simulink model "SWC_FDC_type"  (R2021b)
settings: Solver=FixedStepDiscrete  StartTime=0.0  StopTime=10.0  FixedStep=0.001  RelTol=1e-3
values from neighbouring files (symbols this model uses):
  C_TASK_5MS_S = (	C_TICK_TIME_S      	)    [vcu_local_hdr.m]
  DID_VCUKey = uint16(0x0202)    [vcu_local_hdr.m]
  DID_XWD = uint16(513)    [vcu_local_hdr.m]
  DIDLen_APPPedalZP = uint16(3)    [vcu_local_hdr.m]
  DIDLen_APSFunConfig = uint16(16)    [vcu_local_hdr.m]
  DIDLen_AutoLock = uint16(1)    [vcu_local_hdr.m]
  DIDLen_AutoWipHSpdEN = uint16(1)    [vcu_local_hdr.m]
  DIDLen_DKCKey = uint16(8)    [vcu_local_hdr.m]
  DIDLen_DRLDis = uint16(1)    [vcu_local_hdr.m]
  DIDLen_DynoMode = uint16(1)    [vcu_local_hdr.m]
  DIDLen_FMHTimer = uint16(1)    [vcu_local_hdr.m]
  DIDLen_LFLowPresThre = uint16(1)    [vcu_local_hdr.m]
  DIDLen_LFSensorID = uint16(4)    [vcu_local_hdr.m]
  DIDLen_LRLowPresThre = uint16(1)    [vcu_local_hdr.m]
  DIDLen_LRSensorID = uint16(4)    [vcu_local_hdr.m]
  DIDLen_NVMPedalZP = uint16(3)    [vcu_local_hdr.m]
  DIDLen_RFLowPresThre = uint16(1)    [vcu_local_hdr.m]
  DIDLen_RFSensorID = uint16(4)    [vcu_local_hdr.m]
  DIDLen_RRLowPresThre = uint16(1)    [vcu_local_hdr.m]
  DIDLen_RRSensorID = uint16(4)    [vcu_local_hdr.m]
  DIDLen_SensorMode = uint16(1)    [vcu_local_hdr.m]
  DIDLen_TireSize = uint16(16)    [vcu_local_hdr.m]
  DIDLen_TPMSLearnSta = uint16(1)    [vcu_local_hdr.m]
  DIDLen_TurnLampFLThreCurr = uint16(1)    [vcu_local_hdr.m]
  DIDLen_TurnLampFRThreCurr = uint16(1)    [vcu_local_hdr.m]
  DIDLen_TurnLampRLThreCurr = uint16(1)    [vcu_local_hdr.m]
  DIDLen_TurnLampRRThreCurr = uint16(1)    [vcu_local_hdr.m]
  DIDLen_USSConfig = uint16(16)    [vcu_local_hdr.m]
  DIDLen_WhlPres = uint16(4)    [vcu_local_hdr.m]
  DIDLen_WhlSensorBattSta = uint16(1)    [vcu_local_hdr.m]
  DIDLen_WhlTmp = uint16(4)    [vcu_local_hdr.m]
  DIDLen_WipRLSCmdCutFilter = uint16(1)    [vcu_local_hdr.m]
  DIDLen_WipRLSCmdHoldFilter = uint16(1)    [vcu_local_hdr.m]
  DIDLen_XWDMode = uint16(1)    [vcu_local_hdr.m]
  DIDNum_APPPedalZP = uint16(0x0206)    [vcu_local_hdr.m]
  DIDNum_APSFunConfig = uint16(0x0903)    [vcu_local_hdr.m]
  DIDNum_AutoLock = uint16(0x0306)    [vcu_local_hdr.m]
  DIDNum_AutoWipHSpdEN = uint16(0x0308)    [vcu_local_hdr.m]
  DIDNum_DKCKey = uint16(0x0202)    [vcu_local_hdr.m]
  DIDNum_DRLDis = uint16(0x0307)    [vcu_local_hdr.m]
  DIDNum_DynoMode = uint16(0x0203)    [vcu_local_hdr.m]
  DIDNum_FMHTimer = uint16(0x0305)    [vcu_local_hdr.m]
  DIDNum_LFLowPresThre = uint16(0x0B08)    [vcu_local_hdr.m]
  DIDNum_LFSensorID = uint16(0x0B01)    [vcu_local_hdr.m]
  DIDNum_LRLowPresThre = uint16(0x0B0A)    [vcu_local_hdr.m]
  DIDNum_LRSensorID = uint16(0x0B03)    [vcu_local_hdr.m]
  DIDNum_NVMPedalZP = uint16(0x0207)    [vcu_local_hdr.m]
  DIDNum_RFLowPresThre = uint16(0x0B09)    [vcu_local_hdr.m]
  DIDNum_RFSensorID = uint16(0x0B02)    [vcu_local_hdr.m]
  DIDNum_RRLowPresThre = uint16(0x0B0B)    [vcu_local_hdr.m]
  DIDNum_RRSensorID = uint16(0x0B04)    [vcu_local_hdr.m]
  DIDNum_SensorMode = uint16(0x0B0C)    [vcu_local_hdr.m]
  DIDNum_TireSize = uint16(0x0902)    [vcu_local_hdr.m]
  DIDNum_TPMSLearnSta = uint16(0x0B0D)    [vcu_local_hdr.m]
  DIDNum_TurnLampFLThreCurr = uint16(0x0303)    [vcu_local_hdr.m]
  DIDNum_TurnLampFRThreCurr = uint16(0x0301)    [vcu_local_hdr.m]
  DIDNum_TurnLampRLThreCurr = uint16(0x0304)    [vcu_local_hdr.m]
  DIDNum_TurnLampRRThreCurr = uint16(0x0302)    [vcu_local_hdr.m]
  DIDNum_USSConfig = uint16(0x0901)    [vcu_local_hdr.m]
  DIDNum_WhlPres = uint16(0x0B05)    [vcu_local_hdr.m]
  DIDNum_WhlSensorBattSta = uint16(0x0B07)    [vcu_local_hdr.m]
  DIDNum_WhlTmp = uint16(0x0B06)    [vcu_local_hdr.m]
  DIDNum_WipRLSCmdCutFilter = uint16(0x030A)    [vcu_local_hdr.m]
  DIDNum_WipRLSCmdHoldFilter = uint16(0x0309)    [vcu_local_hdr.m]
  DIDNum_XWDMode = uint16(0x0201)    [vcu_local_hdr.m]
  DIDVCUKeyLength = uint16(8)    [vcu_local_hdr.m]
  DTC_10020B = Simulink.Parameter    [DTC_Constant_Definition.m]
  DTC_10020C = Simulink.Parameter    [DTC_Constant_Definition.m]
  DTC_10020D = Simulink.Parameter    [DTC_Constant_Definition.m]
  DTC_10020E = Simulink.Parameter    [DTC_Constant_Definition.m]
  DTC_100210 = Simulink.Parameter    [DTC_Constant_Definition.m]
  DTC_100211 = Simulink.Parameter    [DTC_Constant_Definition.m]
  DTC_100212 = Simulink.Parameter    [DTC_Constant_Definition.m]
  DTC_100213 = Simulink.Parameter    [DTC_Constant_Definition.m]
  DTC_100214 = Simulink.Parameter    [DTC_Constant_Definition.m]
  DTC_100215 = Simulink.Parameter    [DTC_Constant_Definition.m]
  DTC_100216 = Simulink.Parameter    [DTC_Constant_Definition.m]
  DTC_100217 = Simulink.Parameter    [DTC_Constant_Definition.m]
  DTC_100218 = Simulink.Parameter    [DTC_Constant_Definition.m]
  DTC_100219 = Simulink.Parameter    [DTC_Constant_Definition.m]
  DTC_10021A = Simulink.Parameter    [DTC_Constant_Definition.m]
  DTC_10021B = Simulink.Parameter    [DTC_Constant_Definition.m]
  DTC_10021C = Simulink.Parameter    [DTC_Constant_Definition.m]
  DTC_10021D = Simulink.Parameter    [DTC_Constant_Definition.m]
  DTC_10021E = Simulink.Parameter    [DTC_Constant_Definition.m]
  DTC_100220 = Simulink.Parameter    [DTC_Constant_Definition.m]
  DTC_100221 = Simulink.Parameter    [DTC_Constant_Definition.m]
  DTC_100223 = Simulink.Parameter    [DTC_Constant_Definition.m]
  DTC_100224 = Simulink.Parameter    [DTC_Constant_Definition.m]
  DTC_100225 = Simulink.Parameter    [DTC_Constant_Definition.m]
  DTC_100226 = Simulink.Parameter    [DTC_Constant_Definition.m]
  DTC_100227 = Simulink.Parameter    [DTC_Constant_Definition.m]
  DTC_100242 = Simulink.Parameter    [DTC_Constant_Definition.m]
  DTC_100243 = Simulink.Parameter    [DTC_Constant_Definition.m]
  DTC_100244 = Simulink.Parameter    [DTC_Constant_Definition.m]
  DTC_100247 = Simulink.Parameter    [DTC_Constant_Definition.m]
  DTC_100248 = Simulink.Parameter    [DTC_Constant_Definition.m]
  DTC_100249 = Simulink.Parameter    [DTC_Constant_Definition.m]
  DTC_100250 = Simulink.Parameter    [DTC_Constant_Definition.m]
  DTC_100251 = Simulink.Parameter    [DTC_Constant_Definition.m]
  DTC_100252 = Simulink.Parameter    [DTC_Constant_Definition.m]
  DTC_100A10 = Simulink.Parameter    [DTC_Constant_Definition.m]
  DTC_100A12 = Simulink.Parameter    [DTC_Constant_Definition.m]
  DTC_100A16 = Simulink.Parameter    [DTC_Constant_Definition.m]
  DTC_100A17 = Simulink.Parameter    [DTC_Constant_Definition.m]
  DTC_100A18 = Simulink.Parameter    [DTC_Constant_Definition.m]
  DTC_100A19 = Simulink.Parameter    [DTC_Constant_Definition.m]
  DTC_500B01 = Simulink.Parameter    [DTC_Constant_Definition.m]
  DTC_500B02 = Simulink.Parameter    [DTC_Constant_Definition.m]
  DTC_500B03 = Simulink.Parameter    [DTC_Constant_Definition.m]
  DTC_500B04 = Simulink.Parameter    [DTC_Constant_Definition.m]
  DTC_500B05 = Simulink.Parameter    [DTC_Constant_Definition.m]
  DTC_500B06 = Simulink.Parameter    [DTC_Constant_Definition.m]
  DTC_500B07 = Simulink.Parameter    [DTC_Constant_Definition.m]
  DTC_500B08 = Simulink.Parameter    [DTC_Constant_Definition.m]
  DTC_500B09 = Simulink.Parameter    [DTC_Constant_Definition.m]
  DTC_500B0A = Simulink.Parameter    [DTC_Constant_Definition.m]
  DTC_500B0B = Simulink.Parameter    [DTC_Constant_Definition.m]
  DTC_500B0C = Simulink.Parameter    [DTC_Constant_Definition.m]
  DTC_500B0D = Simulink.Parameter    [DTC_Constant_Definition.m]
  ... (+93 more)
undefined symbols (not defined in the file or in its folder): f32_ApsOutVehSpdSig, KHAL_CANBusOffDebounce_cnt, KHAL_CANBusOffDebounce_s, KHAL_DKCDecryptEnable_flg_ovrdflg, KHAL_DKCDecryptEnable_flg_ovrdval, KHAL_RandomNumberY1_enum, KHAL_RandomNumberY2_enum, KHAL_RandomNumberY_ovrdflg, KHAL_TPMSRESBUTT_flg_ovrdflg, KHAL_TPMSRESBUTT_flg_ovrdval, KINP_ReadVinCode_flg, KTQD_DefaultRegenMode_enum, R_DIDWriteCDD_CSOP_DIDSet_APPPedalZP, R_DIDWriteCDD_CSOP_DIDSet_APSFunConfig, R_DIDWriteCDD_CSOP_DIDSet_AutoLock, R_DIDWriteCDD_CSOP_DIDSet_AutoWipHSpdEN, R_DIDWriteCDD_CSOP_DIDSet_DKCKey, R_DIDWriteCDD_CSOP_DIDSet_DRLDis, R_DIDWriteCDD_CSOP_DIDSet_DynoMode, R_DIDWriteCDD_CSOP_DIDSet_FMHTimer, R_DIDWriteCDD_CSOP_DIDSet_LFLowPresThre, R_DIDWriteCDD_CSOP_DIDSet_LFSensorID, R_DIDWriteCDD_CSOP_DIDSet_LRLowPresThre, R_DIDWriteCDD_CSOP_DIDSet_LRSensorID, R_DIDWriteCDD_CSOP_DIDSet_NVMPedalZP, R_DIDWriteCDD_CSOP_DIDSet_RFLowPresThre, R_DIDWriteCDD_CSOP_DIDSet_RFSensorID, R_DIDWriteCDD_CSOP_DIDSet_RRLowPresThre, R_DIDWriteCDD_CSOP_DIDSet_RRSensorID, R_DIDWriteCDD_CSOP_DIDSet_SensorMode, R_DIDWriteCDD_CSOP_DIDSet_TireSize, R_DIDWriteCDD_CSOP_DIDSet_TPMSLearnSta, R_DIDWriteCDD_CSOP_DIDSet_TurnLampFLThreCurr, R_DIDWriteCDD_CSOP_DIDSet_TurnLampFRThreCurr, R_DIDWriteCDD_CSOP_DIDSet_TurnLampRLThreCurr, R_DIDWriteCDD_CSOP_DIDSet_TurnLampRRThreCurr, R_DIDWriteCDD_CSOP_DIDSet_USSConfig, R_DIDWriteCDD_CSOP_DIDSet_WhlPres, R_DIDWriteCDD_CSOP_DIDSet_WhlSensorBattSta, R_DIDWriteCDD_CSOP_DIDSet_WhlTmp, R_DIDWriteCDD_CSOP_DIDSet_WipRLSCmdCutFilter, R_DIDWriteCDD_CSOP_DIDSet_WipRLSCmdHoldFilter, R_DIDWriteCDD_CSOP_DIDSet_XWDMode, R_E2E_CAN3_VCU1_CSOP_Write_CAN3_VCU1, R_E2E_CAN3_VCU1_toNIDEC_CSOP_Write_CAN3_VCU1_toNIDEC ... (+128)
libraries: simulink x246, FVT_lib x139, hcu_lib x31, hdlsllib x11, app x1, halin x1, halout x1, matrix_library x1, inp x1, outp x1
(part 1 of 13)
settings Model: DataDictionary=APPTypes.sldd  Creator=FVT23010  LastModifiedBy=FVT22115
settings DataIOCC: SaveFormat=StructureWithTime
settings OptimizationCC: DefaultParameterBehavior=Inlined  EnhancedBackFolding=on  PassReuseOutputArgsAs=Individual arguments  ZeroExternalMemoryAtStartup=off  ZeroInternalMemoryAtStartup=off  OptimizeBlockOrder=speed  DifferentSizesBufferReuse=on  OptimizationCustomize=off  EfficientTunableParamExpr=on
settings DebuggingCC: ParameterTunabilityLossMsg=error
settings HardwareCC: ProdBitPerPointer=32  ProdBitPerSizeT=32  ProdBitPerPtrDiffT=32  ProdLargestAtomicInteger=Long  ProdLargestAtomicFloat=Double  ProdWordSize=32  ProdLongLongMode=on  ProdHWDeviceType=ARM Compatible->ARM Cortex-M
settings ModelReferenceCC: ModelReferenceNumInstancesAllowed=Single
settings SFSimCC: MATLABDynamicMemAlloc=off
settings RTWCC: Description=AUTOSAR  SystemTargetFile=autosar.tlc  GenCodeOnly=on  TemplateMakefile=ert_default_tmf  PortableWordSizes=on
settings CodeAppCC: ForceParamTrailComments=on  IgnoreCustomStorageClasses=off  OperatorAnnotations=on  SimulinkDataObjDesc=on  SFDataObjDesc=on  InsertBlockDesc=on
settings STFCustomTargetCC: TargetLangStandard=C99 (ISO)  MultiwordLength=256  ParMdlRefBuildCompliant=on  CompOptLevelCompliant=on  IncludeMdlTerminateFcn=off  CombineOutputUpdateFcns=on  SuppressErrorStatus=on  ERTCustomFileBanners=on  SupportNonFinite=off  SupportComplex=off  SupportContinuousTime=off  SupportNonInlinedSFcns=off  RemoveResetFunc=on  MATLABClassNameForMDSCustomization=Simulink.SoftwareTarget.ERTCustomization  AutosarCompliant=on  GRTInterface=off  UseToolchainInfoCompliant=on  LookupTableObjectStructAxisOrder=2,1,3,4,...  LUTObjectStructOrderEvenSpacing=Size,Table,Breakpoints  SystemTargetFile=autosar.tlc
settings ERTTargetCC: TargetLangStandard=C99 (ISO)  ConcurrentExecutionCompliant=off  IncludeMdlTerminateFcn=off  SuppressErrorStatus=on  SupportNonFinite=off  SupportComplex=off  ModelStepFunctionPrototypeControlCompliant=off  CPPClassGenCompliant=off  AutosarCompliant=on  LookupTableObjectStructAxisOrder=2,1,3,4,...  LUTObjectStructOrderEvenSpacing=Size,Table,Breakpoints  GenerateASAP2=on  InlinedParameterPlacement=NonHierarchical  ERTCustomFileTemplate=example_file_process.tlc  ConvertIfToSwitch=off  SuppressUnreachableDefaultCases=off  BooleanTrueId=true_MatlabRTW  BooleanFalseId=false_MatlabRTW

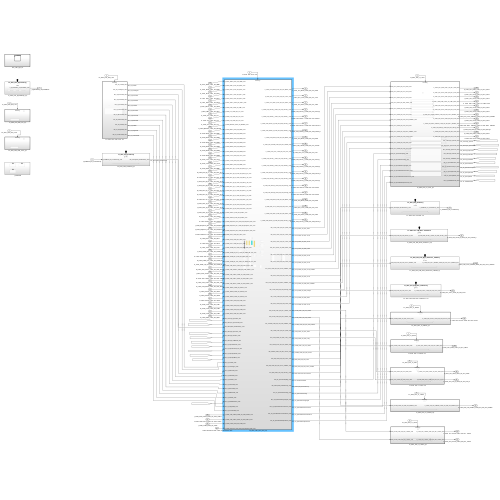
[thumbnail: Simulink's stored preview of the top-level diagram]
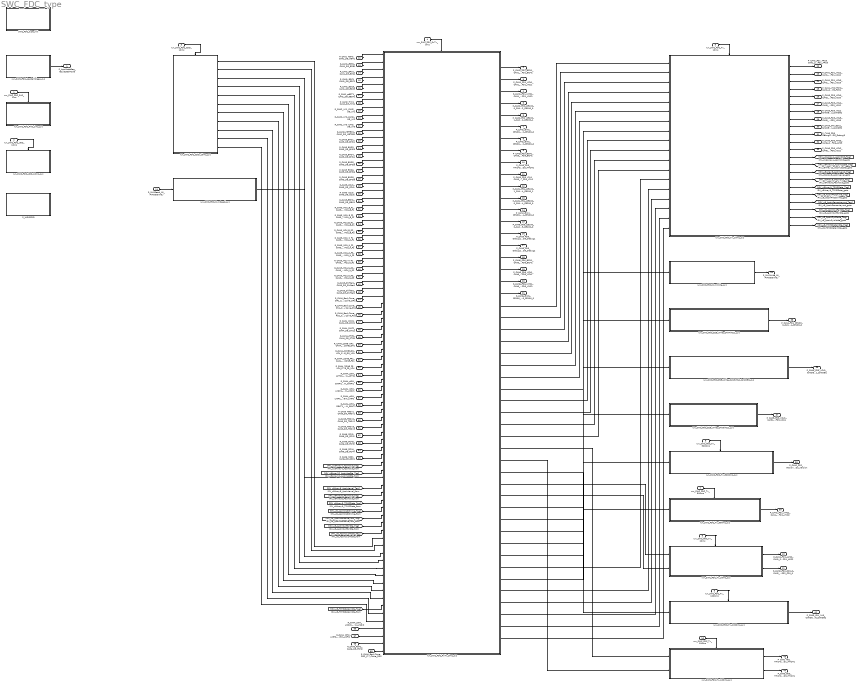
== system SWC_FDC_type ==
  run_SWC_FDC_PAS_1ms : Inport  SampleTime=0.001  OutputFunctionCall=on
  run_SWC_FDC_UDS_10ms : Inport  Port=2  SampleTime=0.01  OutputFunctionCall=on
  run_SWC_FDC_CDD_10ms : Inport  Port=3  SampleTime=0.01  OutputFunctionCall=on
  run_SWC_FDC_RxTx_5ms : Inport  Port=4  SampleTime=0.005  OutputFunctionCall=on
  run_SWC_FDC_Tx_10ms : Inport  Port=5  SampleTime=0.01  OutputFunctionCall=on
  run_SWC_FDC_Tx_5000ms : Inport  Port=6  SampleTime=5  OutputFunctionCall=on
  run_SWC_FDC_Tx_500ms : Inport  Port=7  SampleTime=0.5  OutputFunctionCall=on
  run_SWC_FDC_Tx_20ms : Inport  Port=8  SampleTime=0.02  OutputFunctionCall=on
  run_SWC_FDC_Tx_1000ms : Inport  Port=9  SampleTime=1  OutputFunctionCall=on
  run_SWC_FDC_Tx_100ms : Inport  Port=10  SampleTime=0.1  OutputFunctionCall=on
  R_NVMRead_NV_FVTDataArray : Inport  Port=11  OutDataTypeStr=uint8  PortDimensions=256
  R_CAN1_ABM1_CAN1_SG_ABM1 : Inport  Port=12  OutDataTypeStr=Bus: DT_CAN1_SG_ABM1  PortDimensions=1  BusOutputAsStruct=on
  R_CAN1_EPB1_CAN1_SG_EPB1 : Inport  Port=13  OutDataTypeStr=Bus: DT_CAN1_SG_EPB1  PortDimensions=1  BusOutputAsStruct=on
  R_CAN1_EPS1_CAN1_SG_EPS1 : Inport  Port=14  OutDataTypeStr=Bus: DT_CAN1_SG_EPS1  PortDimensions=1  BusOutputAsStruct=on
  R_CAN1_ESC1_CAN1_SG_ESC1 : Inport  Port=15  OutDataTypeStr=Bus: DT_CAN1_SG_ESC1  PortDimensions=1  BusOutputAsStruct=on
  R_CAN1_ESC5_CAN1_SG_ESC5 : Inport  Port=16  OutDataTypeStr=Bus: DT_CAN1_SG_ESC5  PortDimensions=1  BusOutputAsStruct=on
  R_CAN1_eBST1_CAN1_SG_eBST1 : Inport  Port=17  OutDataTypeStr=Bus: DT_CAN1_SG_eBST1  PortDimensions=1  BusOutputAsStruct=on
  R_CAN2_HMI1_CAN2_SG_HMI1 : Inport  Port=18  OutDataTypeStr=Bus: DT_CAN2_SG_HMI1  PortDimensions=1  BusOutputAsStruct=on
  R_CAN2_IVI1_CAN2_SG_IVI1 : Inport  Port=19  OutDataTypeStr=Bus: DT_CAN2_SG_IVI1  PortDimensions=1  BusOutputAsStruct=on
  R_CAN2_IVI2_CAN2_SG_IVI2 : Inport  Port=20  OutDataTypeStr=Bus: DT_CAN2_SG_IVI2  PortDimensions=1  BusOutputAsStruct=on
  R_CAN2_IVI3_CAN2_SG_IVI3 : Inport  Port=21  OutDataTypeStr=Bus: DT_CAN2_SG_IVI3  PortDimensions=1  BusOutputAsStruct=on
  R_CAN2_METER1_CAN2_SG_METER1 : Inport  Port=22  OutDataTypeStr=Bus: DT_CAN2_SG_METER1  PortDimensions=1  BusOutputAsStruct=on
  R_CAN3_BMS1_CAN3_SG_BMS1 : Inport  Port=23  OutDataTypeStr=Bus: DT_CAN3_SG_BMS1  PortDimensions=1  BusOutputAsStruct=on
  R_CAN3_BMS3_CAN3_SG_BMS3 : Inport  Port=24  OutDataTypeStr=Bus: DT_CAN3_SG_BMS3  PortDimensions=1  BusOutputAsStruct=on
  R_CAN3_BMS4_CAN3_SG_BMS4 : Inport  Port=25  OutDataTypeStr=Bus: DT_CAN3_SG_BMS4  PortDimensions=1  BusOutputAsStruct=on
  R_CAN3_BMS5_CAN3_SG_BMS5 : Inport  Port=26  OutDataTypeStr=Bus: DT_CAN3_SG_BMS5  PortDimensions=1  BusOutputAsStruct=on
  R_CAN3_BMS6_CAN3_SG_BMS6 : Inport  Port=27  OutDataTypeStr=Bus: DT_CAN3_SG_BMS6  PortDimensions=1  BusOutputAsStruct=on
  R_CAN3_BMS8_CAN3_SG_BMS8 : Inport  Port=28  OutDataTypeStr=Bus: DT_CAN3_SG_BMS8  PortDimensions=1  BusOutputAsStruct=on
  R_CAN3_CCU1_CAN3_SG_CCU1 : Inport  Port=29  OutDataTypeStr=Bus: DT_CAN3_SG_CCU1  PortDimensions=1  BusOutputAsStruct=on
  R_CAN3_CCU2_CAN3_SG_CCU2 : Inport  Port=30  OutDataTypeStr=Bus: DT_CAN3_SG_CCU2  PortDimensions=1  BusOutputAsStruct=on
  R_CAN3_EBM1_CAN3_SG_EBM1 : Inport  Port=31  OutDataTypeStr=Bus: DT_CAN3_SG_EBM1  PortDimensions=1  BusOutputAsStruct=on
  R_CAN3_MCU_B_F1_CAN3_SG_MCU_B_F1 : Inport  Port=32  OutDataTypeStr=Bus: DT_CAN3_SG_MCU_B_F1  PortDimensions=1  BusOutputAsStruct=on
  R_CAN3_MCU_B_F2_CAN3_SG_MCU_B_F2 : Inport  Port=33  OutDataTypeStr=Bus: DT_CAN3_SG_MCU_B_F2  PortDimensions=1  BusOutputAsStruct=on
  R_CAN3_MCU_B_R1_CAN3_SG_MCU_B_R1 : Inport  Port=34  OutDataTypeStr=Bus: DT_CAN3_SG_MCU_B_R1  PortDimensions=1  BusOutputAsStruct=on
  R_CAN3_MCU_B_R2_CAN3_SG_MCU_B_R2 : Inport  Port=35  OutDataTypeStr=Bus: DT_CAN3_SG_MCU_B_R2  PortDimensions=1  BusOutputAsStruct=on
  R_CAN3_MCU_N_F1_CAN3_SG_MCU_N_F1 : Inport  Port=36  OutDataTypeStr=Bus: DT_CAN3_SG_MCU_N_F1  PortDimensions=1  BusOutputAsStruct=on
  R_CAN3_MCU_N_F2_CAN3_SG_MCU_N_F2 : Inport  Port=37  OutDataTypeStr=Bus: DT_CAN3_SG_MCU_N_F2  PortDimensions=1  BusOutputAsStruct=on
  R_CAN3_MCU_N_F3_CAN3_SG_MCU_N_F3 : Inport  Port=38  OutDataTypeStr=Bus: DT_CAN3_SG_MCU_N_F3  PortDimensions=1  BusOutputAsStruct=on
  R_CAN3_MCU_N_R1_CAN3_SG_MCU_N_R1 : Inport  Port=39  OutDataTypeStr=Bus: DT_CAN3_SG_MCU_N_R1  PortDimensions=1  BusOutputAsStruct=on
  R_CAN3_MCU_N_R2_CAN3_SG_MCU_N_R2 : Inport  Port=40  OutDataTypeStr=Bus: DT_CAN3_SG_MCU_N_R2  PortDimensions=1  BusOutputAsStruct=on
  R_CAN3_MCU_N_R3_CAN3_SG_MCU_N_R3 : Inport  Port=41  OutDataTypeStr=Bus: DT_CAN3_SG_MCU_N_R3  PortDimensions=1  BusOutputAsStruct=on
  R_CAN3_Shifter1_CAN3_SG_Shifter1 : Inport  Port=42  OutDataTypeStr=Bus: DT_CAN3_SG_Shifter1  PortDimensions=1  BusOutputAsStruct=on
  R_CAN3_Shifter2_CAN3_SG_Shifter2 : Inport  Port=43  OutDataTypeStr=Bus: DT_CAN3_SG_Shifter2  PortDimensions=1  BusOutputAsStruct=on
  R_CAN4_BodyZone_DR1_CAN4_SG_BodyZone_DR1 : Inport  Port=44  OutDataTypeStr=Bus: DT_CAN4_SG_BodyZone_DR1  PortDimensions=1  BusOutputAsStruct=on
  R_CAN4_BodyZone_PS1_CAN4_SG_BodyZone_PS1 : Inport  Port=45  OutDataTypeStr=Bus: DT_CAN4_SG_BodyZone_PS1  PortDimensions=1  BusOutputAsStruct=on
  R_CAN4_BodyZone_PS2_CAN4_SG_BodyZone_PS2 : Inport  Port=46  OutDataTypeStr=Bus: DT_CAN4_SG_BodyZone_PS2  PortDimensions=1  BusOutputAsStruct=on
  R_CAN4_DKC1_CAN4_SG_DKC1 : Inport  Port=47  OutDataTypeStr=Bus: DT_CAN4_SG_DKC1  PortDimensions=1  BusOutputAsStruct=on
  R_CAN4_DKC2_CAN4_SG_DKC2 : Inport  Port=48  OutDataTypeStr=Bus: DT_CAN4_SG_DKC2  PortDimensions=1  BusOutputAsStruct=on
  R_CAN4_PTG1_CAN4_SG_PTG1 : Inport  Port=49  OutDataTypeStr=Bus: DT_CAN4_SG_PTG1  PortDimensions=1  BusOutputAsStruct=on
  R_CAN4_ZONE_DR1_CAN4_SG_ZONE_DR1 : Inport  Port=50  OutDataTypeStr=Bus: DT_CAN4_SG_ZONE_DR1  PortDimensions=1  BusOutputAsStruct=on
  R_CAN4_ZONE_DR_VCU_CAN4_SG_ZONE_DR_VCU : Inport  Port=51  OutDataTypeStr=Bus: DT_CAN4_SG_ZONE_DR_VCU  PortDimensions=1  BusOutputAsStruct=on
  R_CAN4_ZONE_FR1_CAN4_SG_ZONE_FR1 : Inport  Port=52  OutDataTypeStr=Bus: DT_CAN4_SG_ZONE_FR1  PortDimensions=1  BusOutputAsStruct=on
  R_CAN4_ZONE_FR_VCU_CAN4_SG_ZONE_FR_VCU : Inport  Port=53  OutDataTypeStr=Bus: DT_CAN4_SG_ZONE_FR_VCU  PortDimensions=1  BusOutputAsStruct=on
  R_CAN4_zGW_APTC1_CAN4_SG_zGW_APTC1 : Inport  Port=54  OutDataTypeStr=Bus: DT_CAN4_SG_zGW_APTC1  PortDimensions=1  BusOutputAsStruct=on
  R_CAN4_zGW_CANFr1_CAN4_SG_zGW_CANFr1 : Inport  Port=55  OutDataTypeStr=Bus: DT_CAN4_SG_zGW_CANFr1  PortDimensions=1  BusOutputAsStruct=on
  R_CAN4_zGW_LINDr1_CAN4_SG_zGW_LINDr1 : Inport  Port=56  OutDataTypeStr=Bus: DT_CAN4_SG_zGW_LINDr1  PortDimensions=1  BusOutputAsStruct=on
  R_CAN4_zGW_LINFr1_CAN4_SG_zGW_LINFr1 : Inport  Port=57  OutDataTypeStr=Bus: DT_CAN4_SG_zGW_LINFr1  PortDimensions=1  BusOutputAsStruct=on
  R_CAN4_zGW_SEAT1_CAN4_SG_zGW_SEAT1 : Inport  Port=58  OutDataTypeStr=Bus: DT_CAN4_SG_zGW_SEAT1  PortDimensions=1  BusOutputAsStruct=on
  R_CAN5_TBOX1_CAN5_SG_TBOX1 : Inport  Port=59  OutDataTypeStr=Bus: DT_CAN5_SG_TBOX1  PortDimensions=1  BusOutputAsStruct=on
  R_CAN5_TBOX2_CAN5_SG_TBOX2 : Inport  Port=60  OutDataTypeStr=Bus: DT_CAN5_SG_TBOX2  PortDimensions=1  BusOutputAsStruct=on
  R_CAN5_TBOX3_CAN5_SG_TBOX3 : Inport  Port=61  OutDataTypeStr=Bus: DT_CAN5_SG_TBOX3  PortDimensions=1  BusOutputAsStruct=on
  R_CAN6_FCM1_CAN6_SG_FCM1 : Inport  Port=62  OutDataTypeStr=Bus: DT_CAN6_SG_FCM1  PortDimensions=1  BusOutputAsStruct=on
  R_CAN6_FCM3_CAN6_SG_FCM3 : Inport  Port=63  OutDataTypeStr=Bus: DT_CAN6_SG_FCM3  PortDimensions=1  BusOutputAsStruct=on
  R_CAN6_FCM4_CAN6_SG_FCM4 : Inport  Port=64  OutDataTypeStr=Bus: DT_CAN6_SG_FCM4  PortDimensions=1  BusOutputAsStruct=on
  R_CAN6_SRR1_CAN6_SG_SRR1 : Inport  Port=65  OutDataTypeStr=Bus: DT_CAN6_SG_SRR1  PortDimensions=1  BusOutputAsStruct=on
  R_CAN4_zGW_LINDr2_CAN4_SG_zGW_LINDr2 : Inport  Port=66  OutDataTypeStr=Bus: DT_CAN4_SG_zGW_LINDr2  PortDimensions=1  BusOutputAsStruct=on
  R_CAN4_zGW_LINFr2_CAN4_SG_zGW_LINFr2 : Inport  Port=67  OutDataTypeStr=Bus: DT_CAN4_SG_zGW_LINFr2  PortDimensions=1  BusOutputAsStruct=on
  R_CAN6_FCM2_CAN6_SG_FCM2 : Inport  Port=68  OutDataTypeStr=Bus: DT_CAN6_SG_FCM2  PortDimensions=1  BusOutputAsStruct=on
  R_CAN4_BodyZone_DR2_CAN4_SG_BodyZone_DR2 : Inport  Port=69  OutDataTypeStr=Bus: DT_CAN4_SG_BodyZone_DR2  PortDimensions=1  BusOutputAsStruct=on
  P_WDGCDD : Subsystem
  SWC_FDC_type_Init : Subsystem
  run_SWC_FDC_AppCallSleep_sys : Subsystem
  run_SWC_FDC_CDD_10ms_sys : Subsystem
  run_SWC_FDC_E2E_Write_CAN3VCU1_sys : Subsystem
  run_SWC_FDC_E2E_Write_CAN3VCU1_toNIDEC_sys : Subsystem
  run_SWC_FDC_E2E_Write_CAN4VCU1_sys : Subsystem
  run_SWC_FDC_NvmRead_sys : Subsystem
  run_SWC_FDC_NvmWrite_sys : Subsystem
  run_SWC_FDC_PAS_1ms_sys : Subsystem
  run_SWC_FDC_RxTx_5ms_sys : Subsystem
  run_SWC_FDC_Tx_1000ms_sys : Subsystem
  run_SWC_FDC_Tx_100ms_sys : Subsystem
  run_SWC_FDC_Tx_10ms_sys : Subsystem
  run_SWC_FDC_Tx_20ms_sys : Subsystem
  run_SWC_FDC_Tx_5000ms_sys : Subsystem
  run_SWC_FDC_Tx_500ms_sys : Subsystem
  run_SWC_FDC_UDS_10ms_sys : Subsystem
  P_AppModeReq_requestedMode : Outport  OutDataTypeStr=Enum: AppModeRequestType  PortDimensions=1
  P_CAN1_FD1_BCM1_CAN1_SG_FD1_BCM1 : Outport  Port=2  OutDataTypeStr=Bus: DT_CAN1_SG_FD1_BCM1  PortDimensions=1  BusOutputAsStruct=on
  P_CAN1_FD1_VCU1_CAN1_SG_FD1_VCU1 : Outport  Port=3  OutDataTypeStr=Bus: DT_CAN1_SG_FD1_VCU1  PortDimensions=1  BusOutputAsStruct=on
  P_CAN1_FD1_VMC1_CAN1_SG_FD1_VMC1 : Outport  Port=4  OutDataTypeStr=Bus: DT_CAN1_SG_FD1_VMC1  PortDimensions=1  BusOutputAsStruct=on
  P_CAN2_FD2_CE100_0_CAN2_SG_FD2_CE100_0 : Outport  Port=5  OutDataTypeStr=Bus: DT_CAN2_SG_FD2_CE100_0  PortDimensions=1  BusOutputAsStruct=on
  P_CAN2_FD2_CE200_1_CAN2_SG_FD2_CE200_1 : Outport  Port=6  OutDataTypeStr=Bus: DT_CAN2_SG_FD2_CE200_1  PortDimensions=1  BusOutputAsStruct=on
  P_CAN2_GW2_CE100_0_CAN2_SG_GW2_CE100_0 : Outport  Port=7  OutDataTypeStr=Bus: DT_CAN2_SG_GW2_CE100_0  PortDimensions=1  BusOutputAsStruct=on
  P_CAN2_GW2_CE200_0_CAN2_SG_GW2_CE200_0 : Outport  Port=8  OutDataTypeStr=Bus: DT_CAN2_SG_GW2_CE200_0  PortDimensions=1  BusOutputAsStruct=on
  P_CAN3_FD3_BCM1_CAN3_SG_FD3_BCM1 : Outport  Port=9  OutDataTypeStr=Bus: DT_CAN3_SG_FD3_BCM1  PortDimensions=1  BusOutputAsStruct=on
  P_CAN3_FD3_THCM2_CAN3_SG_FD3_THCM2 : Outport  Port=10  OutDataTypeStr=Bus: DT_CAN3_SG_FD3_THCM2  PortDimensions=1  BusOutputAsStruct=on
  P_CAN3_FD3_V2L1_CAN3_SG_FD3_V2L1 : Outport  Port=11  OutDataTypeStr=Bus: DT_CAN3_SG_FD3_V2L1  PortDimensions=1  BusOutputAsStruct=on
  P_CAN4_FD4_CE100_1_CAN4_SG_FD4_CE100_1 : Outport  Port=12  OutDataTypeStr=Bus: DT_CAN4_SG_FD4_CE100_1  PortDimensions=1  BusOutputAsStruct=on
  P_CAN4_FD4_CE200_0_CAN4_SG_FD4_CE200_0 : Outport  Port=13  OutDataTypeStr=Bus: DT_CAN4_SG_FD4_CE200_0  PortDimensions=1  BusOutputAsStruct=on
  P_CAN4_GW4_CE100_0_CAN4_SG_GW4_CE100_0 : Outport  Port=14  OutDataTypeStr=Bus: DT_CAN4_SG_GW4_CE100_0  PortDimensions=1  BusOutputAsStruct=on
  P_CAN5_FD5_CE100_0_CAN5_SG_FD5_CE100_0 : Outport  Port=15  OutDataTypeStr=Bus: DT_CAN5_SG_FD5_CE100_0  PortDimensions=1  BusOutputAsStruct=on
  P_CAN5_FD5_Debug1_CAN5_SG_FD5_Debug1 : Outport  Port=16  OutDataTypeStr=Bus: DT_CAN5_SG_FD5_Debug1  PortDimensions=1  BusOutputAsStruct=on
  P_CAN5_FD5_Debug2_CAN5_SG_FD5_Debug2 : Outport  Port=17  OutDataTypeStr=Bus: DT_CAN5_SG_FD5_Debug2  PortDimensions=1  BusOutputAsStruct=on
  P_CAN6_FD6_BCM1_CAN6_SG_FD6_BCM1 : Outport  Port=18  OutDataTypeStr=Bus: DT_CAN6_SG_FD6_BCM1  PortDimensions=1  BusOutputAsStruct=on
  P_CAN6_FD6_VCU1_CAN6_SG_FD6_VCU1 : Outport  Port=19  OutDataTypeStr=Bus: DT_CAN6_SG_FD6_VCU1  PortDimensions=1  BusOutputAsStruct=on
  P_CAN6_FD6_VMC1_CAN6_SG_FD6_VMC1 : Outport  Port=20  OutDataTypeStr=Bus: DT_CAN6_SG_FD6_VMC1  PortDimensions=1  BusOutputAsStruct=on
  P_CAN6_GW6_CE100_0_CAN6_SG_GW6_CE100_0 : Outport  Port=21  OutDataTypeStr=Bus: DT_CAN6_SG_GW6_CE100_0  PortDimensions=1  BusOutputAsStruct=on
  P_CAN1_FD1_APS3_CAN1_SG_FD1_APS3 : Outport  Port=22  OutDataTypeStr=Bus: DT_CAN1_SG_FD1_APS3  PortDimensions=1  BusOutputAsStruct=on
  P_CAN1_FD1_VCU2_CAN1_SG_FD1_VCU2 : Outport  Port=23  OutDataTypeStr=Bus: DT_CAN1_SG_FD1_VCU2  PortDimensions=1  BusOutputAsStruct=on
  P_CAN1_FD1_VCU3_CAN1_SG_FD1_VCU3 : Outport  Port=24  OutDataTypeStr=Bus: DT_CAN1_SG_FD1_VCU3  PortDimensions=1  BusOutputAsStruct=on
  P_CAN1_VMC_FCM1_CAN1_SG_VMC_FCM1 : Outport  Port=25  OutDataTypeStr=Bus: DT_CAN1_SG_VMC_FCM1  PortDimensions=1  BusOutputAsStruct=on
  P_CAN3_FD3_VCU0_CAN3_SG_FD3_VCU0 : Outport  Port=26  OutDataTypeStr=Bus: DT_CAN3_SG_FD3_VCU0  PortDimensions=1  BusOutputAsStruct=on
  P_CAN3_FD3_VCU2_CAN3_SG_FD3_VCU2 : Outport  Port=27  OutDataTypeStr=Bus: DT_CAN3_SG_FD3_VCU2  PortDimensions=1  BusOutputAsStruct=on
  P_CAN3_FD3_VCU2_toNIDEC_CAN3_SG_FD3_VCU2_toNIDEC : Outport  Port=28  OutDataTypeStr=Bus: DT_CAN3_SG_FD3_VCU2_toNIDEC  PortDimensions=1  BusOutputAsStruct=on
  P_CAN3_FD3_VCU5_CAN3_SG_FD3_VCU5 : Outport  Port=29  OutDataTypeStr=Bus: DT_CAN3_SG_FD3_VCU5  PortDimensions=1  BusOutputAsStruct=on
  P_CAN3_GW_ESC1_toNIDEC_CAN3_SG_GW_ESC1_toNIDEC : Outport  Port=30  OutDataTypeStr=Bus: DT_CAN3_SG_GW_ESC1_toNIDEC  PortDimensions=1  BusOutputAsStruct=on
  P_CAN5_FD5_Debug3_CAN5_SG_FD5_Debug3 : Outport  Port=31  OutDataTypeStr=Bus: DT_CAN5_SG_FD5_Debug3  PortDimensions=1  BusOutputAsStruct=on
  P_CAN6_FD6_APS3_CAN6_SG_FD6_APS3 : Outport  Port=32  OutDataTypeStr=Bus: DT_CAN6_SG_FD6_APS3  PortDimensions=1  BusOutputAsStruct=on
  P_CAN6_FD6_VCU2_CAN6_SG_FD6_VCU2 : Outport  Port=33  OutDataTypeStr=Bus: DT_CAN6_SG_FD6_VCU2  PortDimensions=1  BusOutputAsStruct=on
  P_NVMWrite_NV_FVTDataArray : Outport  Port=34  OutDataTypeStr=uint8  PortDimensions=256
  P_CAN4_FD4_CE100_0_CAN4_SG_FD4_CE100_0 : Outport  Port=35  OutDataTypeStr=Bus: DT_CAN4_SG_FD4_CE100_0  PortDimensions=1  BusOutputAsStruct=on
  P_CAN3_FD3_VCU1_toNIDEC_CAN3_SG_FD3_VCU1_toNIDEC : Outport  Port=36  OutDataTypeStr=Bus: DT_CAN3_SG_FD3_VCU1_toNIDEC  PortDimensions=1  BusOutputAsStruct=on
  P_CAN3_FD3_VCU1_CAN3_SG_FD3_VCU1 : Outport  Port=37  OutDataTypeStr=Bus: DT_CAN3_SG_FD3_VCU1  PortDimensions=1  BusOutputAsStruct=on
  P_CAN2_FD2_Version_CAN2_SG_FD2_Version : Outport  Port=38  OutDataTypeStr=Bus: DT_CAN2_SG_FD2_Version  PortDimensions=1  BusOutputAsStruct=on
  P_CAN1_FD1_VMC2_CAN1_SG_FD1_VMC2 : Outport  Port=39  OutDataTypeStr=Bus: DT_CAN1_SG_FD1_VMC2  PortDimensions=1  BusOutputAsStruct=on
  P_CAN1_FD1_APS2_CAN1_SG_FD1_APS2 : Outport  Port=40  OutDataTypeStr=Bus: DT_CAN1_SG_FD1_APS2  PortDimensions=1  BusOutputAsStruct=on
  P_CAN2_FD2_C20_0_CAN2_SG_FD2_C20_0 : Outport  Port=41  OutDataTypeStr=Bus: DT_CAN2_SG_FD2_C20_0  PortDimensions=1  BusOutputAsStruct=on
  P_CAN3_GW_IVI6_toNIDEC_CAN3_SG_GW_IVI6_toNIDEC : Outport  Port=42  OutDataTypeStr=Bus: DT_CAN3_SG_GW_IVI6_toNIDEC  PortDimensions=1  BusOutputAsStruct=on
  P_CAN1_FD1_THCM1_CAN1_SG_FD1_THCM1 : Outport  Port=43  OutDataTypeStr=Bus: DT_CAN1_SG_FD1_THCM1  PortDimensions=1  BusOutputAsStruct=on
  P_CAN3_FD3_THCM1_CAN3_SG_FD3_THCM1 : Outport  Port=44  OutDataTypeStr=Bus: DT_CAN3_SG_FD3_THCM1  PortDimensions=1  BusOutputAsStruct=on
  wires:
  run_SWC_FDC_AppCallSleep_sys/1(P_AppModeReq_requestedMode_write) -> P_AppModeReq_requestedMode/1
  R_NVMRead_NV_FVTDataArray/1 -> run_SWC_FDC_NvmRead_sys/1(R_NVMRead_NV_FVTDataArray_read)
  R_CAN1_ABM1_CAN1_SG_ABM1/1 -> run_SWC_FDC_RxTx_5ms_sys/1(R_CAN1_ABM1_CAN1_SG_ABM1_read)
  R_CAN1_EPB1_CAN1_SG_EPB1/1 -> run_SWC_FDC_RxTx_5ms_sys/2(R_CAN1_EPB1_CAN1_SG_EPB1_read)
  R_CAN1_EPS1_CAN1_SG_EPS1/1 -> run_SWC_FDC_RxTx_5ms_sys/3(R_CAN1_EPS1_CAN1_SG_EPS1_read)
  R_CAN1_ESC1_CAN1_SG_ESC1/1 -> run_SWC_FDC_RxTx_5ms_sys/4(R_CAN1_ESC1_CAN1_SG_ESC1_read)
  R_CAN1_ESC5_CAN1_SG_ESC5/1 -> run_SWC_FDC_RxTx_5ms_sys/5(R_CAN1_ESC5_CAN1_SG_ESC5_read)
  R_CAN1_eBST1_CAN1_SG_eBST1/1 -> run_SWC_FDC_RxTx_5ms_sys/6(R_CAN1_eBST1_CAN1_SG_eBST1_read)
  R_CAN2_HMI1_CAN2_SG_HMI1/1 -> run_SWC_FDC_RxTx_5ms_sys/7(R_CAN2_HMI1_CAN2_SG_HMI1_read)
  R_CAN2_IVI1_CAN2_SG_IVI1/1 -> run_SWC_FDC_RxTx_5ms_sys/8(R_CAN2_IVI1_CAN2_SG_IVI1_read)
  R_CAN2_IVI2_CAN2_SG_IVI2/1 -> run_SWC_FDC_RxTx_5ms_sys/9(R_CAN2_IVI2_CAN2_SG_IVI2_read)
  R_CAN2_IVI3_CAN2_SG_IVI3/1 -> run_SWC_FDC_RxTx_5ms_sys/10(R_CAN2_IVI3_CAN2_SG_IVI3_read)
  R_CAN2_METER1_CAN2_SG_METER1/1 -> run_SWC_FDC_RxTx_5ms_sys/11(R_CAN2_METER1_CAN2_SG_METER1_read)
  R_CAN3_BMS1_CAN3_SG_BMS1/1 -> run_SWC_FDC_RxTx_5ms_sys/12(R_CAN3_BMS1_CAN3_SG_BMS1_read)
  R_CAN3_BMS3_CAN3_SG_BMS3/1 -> run_SWC_FDC_RxTx_5ms_sys/13(R_CAN3_BMS3_CAN3_SG_BMS3_read)
  R_CAN3_BMS4_CAN3_SG_BMS4/1 -> run_SWC_FDC_RxTx_5ms_sys/14(R_CAN3_BMS4_CAN3_SG_BMS4_read)
  R_CAN3_BMS5_CAN3_SG_BMS5/1 -> run_SWC_FDC_RxTx_5ms_sys/15(R_CAN3_BMS5_CAN3_SG_BMS5_read)
  R_CAN3_BMS6_CAN3_SG_BMS6/1 -> run_SWC_FDC_RxTx_5ms_sys/16(R_CAN3_BMS6_CAN3_SG_BMS6_read)
  R_CAN3_BMS8_CAN3_SG_BMS8/1 -> run_SWC_FDC_RxTx_5ms_sys/17(R_CAN3_BMS8_CAN3_SG_BMS8_read)
  R_CAN3_CCU1_CAN3_SG_CCU1/1 -> run_SWC_FDC_RxTx_5ms_sys/18(R_CAN3_CCU1_CAN3_SG_CCU1_read)
  R_CAN3_CCU2_CAN3_SG_CCU2/1 -> run_SWC_FDC_RxTx_5ms_sys/19(R_CAN3_CCU2_CAN3_SG_CCU2_read)
  R_CAN3_EBM1_CAN3_SG_EBM1/1 -> run_SWC_FDC_RxTx_5ms_sys/20(R_CAN3_EBM1_CAN3_SG_EBM1_read)
  R_CAN3_MCU_B_F1_CAN3_SG_MCU_B_F1/1 -> run_SWC_FDC_RxTx_5ms_sys/21(R_CAN3_MCU_B_F1_CAN3_SG_MCU_B_F1_read)
  R_CAN3_MCU_B_F2_CAN3_SG_MCU_B_F2/1 -> run_SWC_FDC_RxTx_5ms_sys/22(R_CAN3_MCU_B_F2_CAN3_SG_MCU_B_F2_read)
  R_CAN3_MCU_B_R1_CAN3_SG_MCU_B_R1/1 -> run_SWC_FDC_RxTx_5ms_sys/23(R_CAN3_MCU_B_R1_CAN3_SG_MCU_B_R1_read)
  R_CAN3_MCU_B_R2_CAN3_SG_MCU_B_R2/1 -> run_SWC_FDC_RxTx_5ms_sys/24(R_CAN3_MCU_B_R2_CAN3_SG_MCU_B_R2_read)
  R_CAN3_MCU_N_F1_CAN3_SG_MCU_N_F1/1 -> run_SWC_FDC_RxTx_5ms_sys/25(R_CAN3_MCU_N_F1_CAN3_SG_MCU_N_F1_read)
  R_CAN3_MCU_N_F2_CAN3_SG_MCU_N_F2/1 -> run_SWC_FDC_RxTx_5ms_sys/26(R_CAN3_MCU_N_F2_CAN3_SG_MCU_N_F2_read)
  R_CAN3_MCU_N_F3_CAN3_SG_MCU_N_F3/1 -> run_SWC_FDC_RxTx_5ms_sys/27(R_CAN3_MCU_N_F3_CAN3_SG_MCU_N_F3_read)
  R_CAN3_MCU_N_R1_CAN3_SG_MCU_N_R1/1 -> run_SWC_FDC_RxTx_5ms_sys/28(R_CAN3_MCU_N_R1_CAN3_SG_MCU_N_R1_read)
  R_CAN3_MCU_N_R2_CAN3_SG_MCU_N_R2/1 -> run_SWC_FDC_RxTx_5ms_sys/29(R_CAN3_MCU_N_R2_CAN3_SG_MCU_N_R2_read)
  R_CAN3_MCU_N_R3_CAN3_SG_MCU_N_R3/1 -> run_SWC_FDC_RxTx_5ms_sys/30(R_CAN3_MCU_N_R3_CAN3_SG_MCU_N_R3_read)
  R_CAN3_Shifter1_CAN3_SG_Shifter1/1 -> run_SWC_FDC_RxTx_5ms_sys/31(R_CAN3_Shifter1_CAN3_SG_Shifter1_read)
  R_CAN3_Shifter2_CAN3_SG_Shifter2/1 -> run_SWC_FDC_RxTx_5ms_sys/32(R_CAN3_Shifter2_CAN3_SG_Shifter2_read)
  R_CAN4_BodyZone_DR1_CAN4_SG_BodyZone_DR1/1 -> run_SWC_FDC_RxTx_5ms_sys/33(R_CAN4_BodyZone_DR1_CAN4_SG_BodyZone_DR1_read)
  R_CAN4_BodyZone_PS1_CAN4_SG_BodyZone_PS1/1 -> run_SWC_FDC_RxTx_5ms_sys/34(R_CAN4_BodyZone_PS1_CAN4_SG_BodyZone_PS1_read)
  R_CAN4_BodyZone_PS2_CAN4_SG_BodyZone_PS2/1 -> run_SWC_FDC_RxTx_5ms_sys/35(R_CAN4_BodyZone_PS2_CAN4_SG_BodyZone_PS2_read)
  R_CAN4_DKC1_CAN4_SG_DKC1/1 -> run_SWC_FDC_RxTx_5ms_sys/36(R_CAN4_DKC1_CAN4_SG_DKC1_read)
  R_CAN4_DKC2_CAN4_SG_DKC2/1 -> run_SWC_FDC_RxTx_5ms_sys/37(R_CAN4_DKC2_CAN4_SG_DKC2_read)
  R_CAN4_PTG1_CAN4_SG_PTG1/1 -> run_SWC_FDC_RxTx_5ms_sys/38(R_CAN4_PTG1_CAN4_SG_PTG1_read)
  R_CAN4_ZONE_DR1_CAN4_SG_ZONE_DR1/1 -> run_SWC_FDC_RxTx_5ms_sys/39(R_CAN4_ZONE_DR1_CAN4_SG_ZONE_DR1_read)
  R_CAN4_ZONE_DR_VCU_CAN4_SG_ZONE_DR_VCU/1 -> run_SWC_FDC_RxTx_5ms_sys/40(R_CAN4_ZONE_DR_VCU_CAN4_SG_ZONE_DR_VCU_read)
  R_CAN4_ZONE_FR1_CAN4_SG_ZONE_FR1/1 -> run_SWC_FDC_RxTx_5ms_sys/41(R_CAN4_ZONE_FR1_CAN4_SG_ZONE_FR1_read)
  R_CAN4_ZONE_FR_VCU_CAN4_SG_ZONE_FR_VCU/1 -> run_SWC_FDC_RxTx_5ms_sys/42(R_CAN4_ZONE_FR_VCU_CAN4_SG_ZONE_FR_VCU_read)
  R_CAN4_zGW_APTC1_CAN4_SG_zGW_APTC1/1 -> run_SWC_FDC_RxTx_5ms_sys/43(R_CAN4_zGW_APTC1_CAN4_SG_zGW_APTC1_read)
  R_CAN4_zGW_CANFr1_CAN4_SG_zGW_CANFr1/1 -> run_SWC_FDC_RxTx_5ms_sys/44(R_CAN4_zGW_CANFr1_CAN4_SG_zGW_CANFr1_read)
  R_CAN4_zGW_LINDr1_CAN4_SG_zGW_LINDr1/1 -> run_SWC_FDC_RxTx_5ms_sys/45(R_CAN4_zGW_LINDr1_CAN4_SG_zGW_LINDr1_read)
  R_CAN4_zGW_LINFr1_CAN4_SG_zGW_LINFr1/1 -> run_SWC_FDC_RxTx_5ms_sys/46(R_CAN4_zGW_LINFr1_CAN4_SG_zGW_LINFr1_read)
  R_CAN4_zGW_SEAT1_CAN4_SG_zGW_SEAT1/1 -> run_SWC_FDC_RxTx_5ms_sys/47(R_CAN4_zGW_SEAT1_CAN4_SG_zGW_SEAT1_read)
  R_CAN5_TBOX1_CAN5_SG_TBOX1/1 -> run_SWC_FDC_RxTx_5ms_sys/48(R_CAN5_TBOX1_CAN5_SG_TBOX1_read)
  R_CAN5_TBOX2_CAN5_SG_TBOX2/1 -> run_SWC_FDC_RxTx_5ms_sys/49(R_CAN5_TBOX2_CAN5_SG_TBOX2_read)
  R_CAN5_TBOX3_CAN5_SG_TBOX3/1 -> run_SWC_FDC_RxTx_5ms_sys/50(R_CAN5_TBOX3_CAN5_SG_TBOX3_read)
  R_CAN6_FCM1_CAN6_SG_FCM1/1 -> run_SWC_FDC_RxTx_5ms_sys/51(R_CAN6_FCM1_CAN6_SG_FCM1_read)
  R_CAN6_FCM3_CAN6_SG_FCM3/1 -> run_SWC_FDC_RxTx_5ms_sys/52(R_CAN6_FCM3_CAN6_SG_FCM3_read)
  R_CAN6_FCM4_CAN6_SG_FCM4/1 -> run_SWC_FDC_RxTx_5ms_sys/53(R_CAN6_FCM4_CAN6_SG_FCM4_read)
  R_CAN6_SRR1_CAN6_SG_SRR1/1 -> run_SWC_FDC_RxTx_5ms_sys/54(R_CAN6_SRR1_CAN6_SG_SRR1_read)
  run_SWC_FDC_RxTx_5ms_sys/1(P_CAN1_FD1_BCM1_CAN1_SG_FD1_BCM1_write) -> P_CAN1_FD1_BCM1_CAN1_SG_FD1_BCM1/1
  run_SWC_FDC_RxTx_5ms_sys/2(P_CAN1_FD1_VCU1_CAN1_SG_FD1_VCU1_write) -> P_CAN1_FD1_VCU1_CAN1_SG_FD1_VCU1/1
  run_SWC_FDC_RxTx_5ms_sys/3(P_CAN1_FD1_VMC1_CAN1_SG_FD1_VMC1_write) -> P_CAN1_FD1_VMC1_CAN1_SG_FD1_VMC1/1
  run_SWC_FDC_RxTx_5ms_sys/4(P_CAN2_FD2_CE100_0_CAN2_SG_FD2_CE100_0_write) -> P_CAN2_FD2_CE100_0_CAN2_SG_FD2_CE100_0/1
  run_SWC_FDC_RxTx_5ms_sys/5(P_CAN2_FD2_CE200_1_CAN2_SG_FD2_CE200_1_write) -> P_CAN2_FD2_CE200_1_CAN2_SG_FD2_CE200_1/1
  run_SWC_FDC_RxTx_5ms_sys/6(P_CAN2_GW2_CE100_0_CAN2_SG_GW2_CE100_0_write) -> P_CAN2_GW2_CE100_0_CAN2_SG_GW2_CE100_0/1
  run_SWC_FDC_RxTx_5ms_sys/7(P_CAN2_GW2_CE200_0_CAN2_SG_GW2_CE200_0_write) -> P_CAN2_GW2_CE200_0_CAN2_SG_GW2_CE200_0/1
  run_SWC_FDC_RxTx_5ms_sys/8(P_CAN3_FD3_BCM1_CAN3_SG_FD3_BCM1_write) -> P_CAN3_FD3_BCM1_CAN3_SG_FD3_BCM1/1
  run_SWC_FDC_RxTx_5ms_sys/9(P_CAN3_FD3_THCM2_CAN3_SG_FD3_THCM2_write) -> P_CAN3_FD3_THCM2_CAN3_SG_FD3_THCM2/1
  run_SWC_FDC_RxTx_5ms_sys/10(P_CAN3_FD3_V2L1_CAN3_SG_FD3_V2L1_write) -> P_CAN3_FD3_V2L1_CAN3_SG_FD3_V2L1/1
  run_SWC_FDC_RxTx_5ms_sys/11(P_CAN4_FD4_CE100_1_CAN4_SG_FD4_CE100_1_write) -> P_CAN4_FD4_CE100_1_CAN4_SG_FD4_CE100_1/1
  run_SWC_FDC_RxTx_5ms_sys/12(P_CAN4_FD4_CE200_0_CAN4_SG_FD4_CE200_0_write) -> P_CAN4_FD4_CE200_0_CAN4_SG_FD4_CE200_0/1
  run_SWC_FDC_RxTx_5ms_sys/13(P_CAN4_GW4_CE100_0_CAN4_SG_GW4_CE100_0_write) -> P_CAN4_GW4_CE100_0_CAN4_SG_GW4_CE100_0/1
  run_SWC_FDC_RxTx_5ms_sys/14(P_CAN5_FD5_CE100_0_CAN5_SG_FD5_CE100_0_write) -> P_CAN5_FD5_CE100_0_CAN5_SG_FD5_CE100_0/1
  run_SWC_FDC_RxTx_5ms_sys/15(P_CAN5_FD5_Debug1_CAN5_SG_FD5_Debug1_write) -> P_CAN5_FD5_Debug1_CAN5_SG_FD5_Debug1/1
  run_SWC_FDC_RxTx_5ms_sys/16(P_CAN5_FD5_Debug2_CAN5_SG_FD5_Debug2_write) -> P_CAN5_FD5_Debug2_CAN5_SG_FD5_Debug2/1
  run_SWC_FDC_RxTx_5ms_sys/17(P_CAN6_FD6_BCM1_CAN6_SG_FD6_BCM1_write) -> P_CAN6_FD6_BCM1_CAN6_SG_FD6_BCM1/1
  run_SWC_FDC_RxTx_5ms_sys/18(P_CAN6_FD6_VCU1_CAN6_SG_FD6_VCU1_write) -> P_CAN6_FD6_VCU1_CAN6_SG_FD6_VCU1/1
  run_SWC_FDC_RxTx_5ms_sys/19(P_CAN6_FD6_VMC1_CAN6_SG_FD6_VMC1_write) -> P_CAN6_FD6_VMC1_CAN6_SG_FD6_VMC1/1
  run_SWC_FDC_RxTx_5ms_sys/20(P_CAN6_GW6_CE100_0_CAN6_SG_GW6_CE100_0_write) -> P_CAN6_GW6_CE100_0_CAN6_SG_GW6_CE100_0/1
  run_SWC_FDC_Tx_10ms_sys/1(P_CAN1_FD1_APS3_CAN1_SG_FD1_APS3_write) -> P_CAN1_FD1_APS3_CAN1_SG_FD1_APS3/1
  run_SWC_FDC_Tx_10ms_sys/2(P_CAN1_FD1_VCU2_CAN1_SG_FD1_VCU2_write) -> P_CAN1_FD1_VCU2_CAN1_SG_FD1_VCU2/1
  run_SWC_FDC_Tx_10ms_sys/3(P_CAN1_FD1_VCU3_CAN1_SG_FD1_VCU3_write) -> P_CAN1_FD1_VCU3_CAN1_SG_FD1_VCU3/1
  run_SWC_FDC_Tx_10ms_sys/4(P_CAN1_VMC_FCM1_CAN1_SG_VMC_FCM1_write) -> P_CAN1_VMC_FCM1_CAN1_SG_VMC_FCM1/1
  run_SWC_FDC_Tx_10ms_sys/5(P_CAN3_FD3_VCU0_CAN3_SG_FD3_VCU0_write) -> P_CAN3_FD3_VCU0_CAN3_SG_FD3_VCU0/1
  run_SWC_FDC_Tx_10ms_sys/6(P_CAN3_FD3_VCU2_CAN3_SG_FD3_VCU2_write) -> P_CAN3_FD3_VCU2_CAN3_SG_FD3_VCU2/1
  run_SWC_FDC_Tx_10ms_sys/7(P_CAN3_FD3_VCU2_toNIDEC_CAN3_SG_FD3_VCU2_toNIDEC_write) -> P_CAN3_FD3_VCU2_toNIDEC_CAN3_SG_FD3_VCU2_toNIDEC/1
  run_SWC_FDC_Tx_10ms_sys/8(P_CAN3_FD3_VCU5_CAN3_SG_FD3_VCU5_write) -> P_CAN3_FD3_VCU5_CAN3_SG_FD3_VCU5/1
  run_SWC_FDC_Tx_10ms_sys/9(P_CAN3_GW_ESC1_toNIDEC_CAN3_SG_GW_ESC1_toNIDEC_write) -> P_CAN3_GW_ESC1_toNIDEC_CAN3_SG_GW_ESC1_toNIDEC/1
  run_SWC_FDC_Tx_10ms_sys/10(P_CAN5_FD5_Debug3_CAN5_SG_FD5_Debug3_write) -> P_CAN5_FD5_Debug3_CAN5_SG_FD5_Debug3/1
  run_SWC_FDC_Tx_10ms_sys/11(P_CAN6_FD6_APS3_CAN6_SG_FD6_APS3_write) -> P_CAN6_FD6_APS3_CAN6_SG_FD6_APS3/1
  run_SWC_FDC_Tx_10ms_sys/12(P_CAN6_FD6_VCU2_CAN6_SG_FD6_VCU2_write) -> P_CAN6_FD6_VCU2_CAN6_SG_FD6_VCU2/1
  run_SWC_FDC_NvmWrite_sys/1(P_NVMWrite_NV_FVTDataArray_write) -> P_NVMWrite_NV_FVTDataArray/1
  run_SWC_FDC_E2E_Write_CAN4VCU1_sys/1(P_CAN4_FD4_CE100_0_CAN4_SG_FD4_CE100_0_write) -> P_CAN4_FD4_CE100_0_CAN4_SG_FD4_CE100_0/1
  run_SWC_FDC_E2E_Write_CAN3VCU1_toNIDEC_sys/1(P_CAN3_FD3_VCU1_toNIDEC_CAN3_SG_FD3_VCU1_toNIDEC_write) -> P_CAN3_FD3_VCU1_toNIDEC_CAN3_SG_FD3_VCU1_toNIDEC/1
  run_SWC_FDC_E2E_Write_CAN3VCU1_sys/1(P_CAN3_FD3_VCU1_CAN3_SG_FD3_VCU1_write) -> P_CAN3_FD3_VCU1_CAN3_SG_FD3_VCU1/1
  run_SWC_FDC_Tx_5000ms_sys/1(P_CAN2_FD2_Version_CAN2_SG_FD2_Version_write) -> P_CAN2_FD2_Version_CAN2_SG_FD2_Version/1
  run_SWC_FDC_Tx_500ms_sys/1(P_CAN1_FD1_VMC2_CAN1_SG_FD1_VMC2_write) -> P_CAN1_FD1_VMC2_CAN1_SG_FD1_VMC2/1
  run_SWC_FDC_Tx_20ms_sys/1(P_CAN1_FD1_APS2_CAN1_SG_FD1_APS2_write) -> P_CAN1_FD1_APS2_CAN1_SG_FD1_APS2/1
  run_SWC_FDC_Tx_20ms_sys/2(P_CAN2_FD2_C20_0_CAN2_SG_FD2_C20_0_write) -> P_CAN2_FD2_C20_0_CAN2_SG_FD2_C20_0/1
  run_SWC_FDC_Tx_1000ms_sys/1(P_CAN3_GW_IVI6_toNIDEC_CAN3_SG_GW_IVI6_toNIDEC_write) -> P_CAN3_GW_IVI6_toNIDEC_CAN3_SG_GW_IVI6_toNIDEC/1
  run_SWC_FDC_Tx_100ms_sys/1(P_CAN1_FD1_THCM1_CAN1_SG_FD1_THCM1_write) -> P_CAN1_FD1_THCM1_CAN1_SG_FD1_THCM1/1
  run_SWC_FDC_Tx_100ms_sys/2(P_CAN3_FD3_THCM1_CAN3_SG_FD3_THCM1_write) -> P_CAN3_FD3_THCM1_CAN3_SG_FD3_THCM1/1
  run_SWC_FDC_CDD_10ms_sys/1(IRV_u8_CTDSW_write) -> run_SWC_FDC_RxTx_5ms_sys/65(IRV_u8_CTDSW_read)  "IRV_u8_CTDSW"
  run_SWC_FDC_CDD_10ms_sys/2(IRV_u8_CrashSignal_write) -> run_SWC_FDC_RxTx_5ms_sys/66(IRV_u8_CrashSignal_read)  "IRV_u8_CrashSignal"
  run_SWC_FDC_CDD_10ms_sys/3(IRV_u8_DrDoorSW_write) -> run_SWC_FDC_RxTx_5ms_sys/67(IRV_u8_DrDoorSW_read)  "IRV_u8_DrDoorSW"
  run_SWC_FDC_CDD_10ms_sys/4(IRV_u8_HazardSW_write) -> run_SWC_FDC_RxTx_5ms_sys/68(IRV_u8_HazardSW_read)  "IRV_u8_HazardSW"
  run_SWC_FDC_CDD_10ms_sys/5(IRV_u8_HoodSW_write) -> run_SWC_FDC_RxTx_5ms_sys/69(IRV_u8_HoodSW_read)  "IRV_u8_HoodSW"
  run_SWC_FDC_CDD_10ms_sys/6(IRV_u8_PsDoorSW_write) -> run_SWC_FDC_RxTx_5ms_sys/70(IRV_u8_PsDoorSW_read)  "IRV_u8_PsDoorSW"
  run_SWC_FDC_CDD_10ms_sys/7(IRV_u8_RLDoorSW_write) -> run_SWC_FDC_RxTx_5ms_sys/71(IRV_u8_RLDoorSW_read)  "IRV_u8_RLDoorSW"
  run_SWC_FDC_CDD_10ms_sys/8(IRV_u8_RRDoorSW_write) -> run_SWC_FDC_RxTx_5ms_sys/72(IRV_u8_RRDoorSW_read)  "IRV_u8_RRDoorSW"
  run_SWC_FDC_CDD_10ms_sys/9(IRV_u8_SeatSW_write) -> run_SWC_FDC_RxTx_5ms_sys/73(IRV_u8_SeatSW_read)  "IRV_u8_SeatSW"
  run_SWC_FDC_CDD_10ms_sys/10(IRV_u8_TailgateSW_write) -> run_SWC_FDC_RxTx_5ms_sys/75(IRV_u8_TailgateSW_read)  "IRV_u8_TailgateSW"
  run_SWC_FDC_CDD_10ms_sys/11(IRV_u8_TrunkHanSW_write) -> run_SWC_FDC_RxTx_5ms_sys/76(IRV_u8_TrunkHanSW_read)  "IRV_u8_TrunkHanSW"
  run_SWC_FDC_NvmRead_sys/1(IRV_u8Array256_NvmReadArray_write) -> run_SWC_FDC_RxTx_5ms_sys/57(IRV_u8Array256_NvmReadArray_read)  "IRV_u8Array256_NvmReadArray"
  run_SWC_FDC_RxTx_5ms_sys/21(IRV_ms10_CAN1_SG_FD1_APS3_write) -> run_SWC_FDC_Tx_10ms_sys/1(IRV_ms10_CAN1_SG_FD1_APS3_read)  "IRV_ms10_CAN1_SG_FD1_APS3"
  run_SWC_FDC_RxTx_5ms_sys/22(IRV_ms10_CAN1_SG_FD1_VCU2_write) -> run_SWC_FDC_Tx_10ms_sys/2(IRV_ms10_CAN1_SG_FD1_VCU2_read)  "IRV_ms10_CAN1_SG_FD1_VCU2"
  run_SWC_FDC_RxTx_5ms_sys/23(IRV_ms10_CAN1_SG_FD1_VCU3_write) -> run_SWC_FDC_Tx_10ms_sys/3(IRV_ms10_CAN1_SG_FD1_VCU3_read)  "IRV_ms10_CAN1_SG_FD1_VCU3"
  run_SWC_FDC_RxTx_5ms_sys/24(IRV_ms10_CAN1_SG_VMC_FCM1_write) -> run_SWC_FDC_Tx_10ms_sys/4(IRV_ms10_CAN1_SG_VMC_FCM1_read)  "IRV_ms10_CAN1_SG_VMC_FCM1"
  run_SWC_FDC_RxTx_5ms_sys/25(IRV_ms10_CAN3_SG_FD3_VCU0_write) -> run_SWC_FDC_Tx_10ms_sys/5(IRV_ms10_CAN3_SG_FD3_VCU0_read)  "IRV_ms10_CAN3_SG_FD3_VCU0"
  run_SWC_FDC_RxTx_5ms_sys/26(IRV_ms10_CAN3_SG_FD3_VCU2_write) -> run_SWC_FDC_Tx_10ms_sys/6(IRV_ms10_CAN3_SG_FD3_VCU2_read)  "IRV_ms10_CAN3_SG_FD3_VCU2"
  run_SWC_FDC_RxTx_5ms_sys/27(IRV_ms10_CAN3_SG_FD3_VCU2_toNIDEC_write) -> run_SWC_FDC_Tx_10ms_sys/7(IRV_ms10_CAN3_SG_FD3_VCU2_toNIDEC_read)  "IRV_ms10_CAN3_SG_FD3_VCU2_toNIDEC"
  run_SWC_FDC_RxTx_5ms_sys/28(IRV_ms10_CAN3_SG_FD3_VCU5_write) -> run_SWC_FDC_Tx_10ms_sys/8(IRV_ms10_CAN3_SG_FD3_VCU5_read)  "IRV_ms10_CAN3_SG_FD3_VCU5"
  run_SWC_FDC_RxTx_5ms_sys/29(IRV_ms10_CAN3_SG_GW_ESC1_toNIDEC_write) -> run_SWC_FDC_Tx_10ms_sys/9(IRV_ms10_CAN3_SG_GW_ESC1_toNIDEC_read)  "IRV_ms10_CAN3_SG_GW_ESC1_toNIDEC"
  run_SWC_FDC_RxTx_5ms_sys/30(IRV_ms10_CAN5_SG_FD5_Debug3_write) -> run_SWC_FDC_Tx_10ms_sys/10(IRV_ms10_CAN5_SG_FD5_Debug3_read)  "IRV_ms10_CAN5_SG_FD5_Debug3"
  run_SWC_FDC_RxTx_5ms_sys/31(IRV_ms10_CAN6_SG_FD6_APS3_write) -> run_SWC_FDC_Tx_10ms_sys/11(IRV_ms10_CAN6_SG_FD6_APS3_read)  "IRV_ms10_CAN6_SG_FD6_APS3"
  run_SWC_FDC_RxTx_5ms_sys/32(IRV_ms10_CAN6_SG_FD6_VCU2_write) -> run_SWC_FDC_Tx_10ms_sys/12(IRV_ms10_CAN6_SG_FD6_VCU2_read)  "IRV_ms10_CAN6_SG_FD6_VCU2"
  run_SWC_FDC_RxTx_5ms_sys/33(IRV_ms100_CAN1_SG_FD1_THCM1_write) -> run_SWC_FDC_Tx_100ms_sys/1(IRV_ms100_CAN1_SG_FD1_THCM1_read)  "IRV_ms100_CAN1_SG_FD1_THCM1"
  run_SWC_FDC_RxTx_5ms_sys/34(IRV_ms100_CAN3_SG_FD3_THCM1_write) -> run_SWC_FDC_Tx_100ms_sys/2(IRV_ms100_CAN3_SG_FD3_THCM1_read)  "IRV_ms100_CAN3_SG_FD3_THCM1"
  run_SWC_FDC_RxTx_5ms_sys/35(IRV_ms1000_CAN3_SG_GW_IVI6_toNIDEC_write) -> run_SWC_FDC_Tx_1000ms_sys/1(IRV_ms1000_CAN3_SG_GW_IVI6_toNIDEC_read)  "IRV_ms1000_CAN3_SG_GW_IVI6_toNIDEC"
  run_SWC_FDC_RxTx_5ms_sys/36(IRV_ms20_CAN1_SG_FD1_APS2_write) -> run_SWC_FDC_Tx_20ms_sys/1(IRV_ms20_CAN1_SG_FD1_APS2_read)  "IRV_ms20_CAN1_SG_FD1_APS2"
  run_SWC_FDC_RxTx_5ms_sys/37(IRV_ms20_CAN2_SG_FD2_C20_0_write) -> run_SWC_FDC_Tx_20ms_sys/2(IRV_ms20_CAN2_SG_FD2_C20_0_read)  "IRV_ms20_CAN2_SG_FD2_C20_0"
  run_SWC_FDC_RxTx_5ms_sys/38(IRV_ms500_CAN1_SG_FD1_VMC2_write) -> run_SWC_FDC_Tx_500ms_sys/1(IRV_ms500_CAN1_SG_FD1_VMC2_read)  "IRV_ms500_CAN1_SG_FD1_VMC2"
  run_SWC_FDC_RxTx_5ms_sys/39(IRV_ms5000_CAN2_SG_FD2_Version_write) -> run_SWC_FDC_Tx_5000ms_sys/1(IRV_ms5000_CAN2_SG_FD2_Version_read)  "IRV_ms5000_CAN2_SG_FD2_Version"
  run_SWC_FDC_RxTx_5ms_sys/40(IRV_E2E_CAN3_SG_FD3_VCU1_write) -> run_SWC_FDC_E2E_Write_CAN3VCU1_sys/1(IRV_E2E_CAN3_SG_FD3_VCU1_read)  "IRV_E2E_CAN3_SG_FD3_VCU1"
  run_SWC_FDC_RxTx_5ms_sys/41(IRV_E2E_CAN3_SG_FD3_VCU1_toNIDEC_write) -> run_SWC_FDC_E2E_Write_CAN3VCU1_toNIDEC_sys/1(IRV_E2E_CAN3_SG_FD3_VCU1_toNIDEC_read)  "IRV_E2E_CAN3_SG_FD3_VCU1_toNIDEC"
  run_SWC_FDC_RxTx_5ms_sys/42(IRV_E2E_CAN4_SG_FD4_CE100_0_write) -> run_SWC_FDC_E2E_Write_CAN4VCU1_sys/1(IRV_E2E_CAN4_SG_FD4_CE100_0_read)  "IRV_E2E_CAN4_SG_FD4_CE100_0"
  run_SWC_FDC_RxTx_5ms_sys/43(IRV_f32_ApsOutVehSpdSig_write) -> run_SWC_FDC_Tx_10ms_sys/13(IRV_f32_ApsOutVehSpdSig_read)  "IRV_f32_ApsOutVehSpdSig"
  run_SWC_FDC_RxTx_5ms_sys/44(IRV_u8Array256_NvmWriteArray_write) -> run_SWC_FDC_NvmWrite_sys/1(IRV_u8Array256_NvmWriteArray_read)  "IRV_u8Array256_NvmWriteArray"
  run_SWC_FDC_RxTx_5ms_sys/45(IRV_u8_ApsOutGearPosnSig_write) -> run_SWC_FDC_Tx_10ms_sys/14(IRV_u8_ApsOutGearPosnSig_read)  "IRV_u8_ApsOutGearPosnSig"
  run_SWC_FDC_RxTx_5ms_sys/46(IRV_u8_ApsOutSendChrgPlugSta_write) -> run_SWC_FDC_Tx_10ms_sys/15(IRV_u8_ApsOutSendChrgPlugSta_read)  "IRV_u8_ApsOutSendChrgPlugSta"
  run_SWC_FDC_RxTx_5ms_sys/47(IRV_u8_ApsOutSetFrSensorOnCmd_write) -> run_SWC_FDC_Tx_10ms_sys/16(IRV_u8_ApsOutSetFrSensorOnCmd_read)  "IRV_u8_ApsOutSetFrSensorOnCmd"
  run_SWC_FDC_RxTx_5ms_sys/48(IRV_u8_ApsOutSetFrSensorSwTOCmd_write) -> run_SWC_FDC_Tx_10ms_sys/17(IRV_u8_ApsOutSetFrSensorSwTOCmd_read)  "IRV_u8_ApsOutSetFrSensorSwTOCmd"
  run_SWC_FDC_RxTx_5ms_sys/49(IRV_u8_ApsOutSetVehSpdTOCmd_write) -> run_SWC_FDC_Tx_10ms_sys/18(IRV_u8_ApsOutSetVehSpdTOCmd_read)  "IRV_u8_ApsOutSetVehSpdTOCmd"
  run_SWC_FDC_Tx_10ms_sys/22(IRV_u8_TPMSDataInSta_write) -> [IRV_u8_TPMSDataInSta_Tag]  "IRV_u8_TPMSDataInSta"
  [IRV_u8_TPMSDataInSta_Tag] -> run_SWC_FDC_RxTx_5ms_sys/74(IRV_u8_TPMSDataInSta_read)
  run_SWC_FDC_Tx_10ms_sys/21(IRV_u8_ApsInSysMode_write) -> [IRV_u8_ApsInSysMode_Tag]  "IRV_u8_ApsInSysMode"
  [IRV_u8_ApsInSysMode_Tag] -> run_SWC_FDC_RxTx_5ms_sys/64(IRV_u8_ApsInSysMode_read)
  run_SWC_FDC_Tx_10ms_sys/20(IRV_u8_ApsInSysFailSta_write) -> [IRV_u8_ApsInSysFailSta_Tag]  "IRV_u8_ApsInSysFailSta"
  [IRV_u8_ApsInSysFailSta_Tag] -> run_SWC_FDC_RxTx_5ms_sys/63(IRV_u8_ApsInSysFailSta_read)
  run_SWC_FDC_Tx_10ms_sys/19(IRV_u8_ApsInSensorLayout_write) -> [IRV_u8_ApsInSensorLayout_Tag]  "IRV_u8_ApsInSensorLayout"
  [IRV_u8_ApsInSensorLayout_Tag] -> run_SWC_FDC_RxTx_5ms_sys/62(IRV_u8_ApsInSensorLayout_read)
  run_SWC_FDC_Tx_10ms_sys/18(IRV_u8_ApsInPASChime_write) -> [IRV_u8_ApsInPASChime_Tag]  "IRV_u8_ApsInPASChime"
  [IRV_u8_ApsInPASChime_Tag] -> run_SWC_FDC_RxTx_5ms_sys/61(IRV_u8_ApsInPASChime_read)
  run_SWC_FDC_Tx_10ms_sys/17(IRV_u8Array9_TPMSData_write) -> [IRV_u8Array9_TPMSData_Tag]  "IRV_u8Array9_TPMSData"
  [IRV_u8Array9_TPMSData_Tag] -> run_SWC_FDC_RxTx_5ms_sys/60(IRV_u8Array9_TPMSData_read)
  run_SWC_FDC_Tx_10ms_sys/16(IRV_u8Array8_PasInDist_write) -> [IRV_u8Array8_PasInDist_Tag]  "IRV_u8Array8_PasInDist"
  [IRV_u8Array8_PasInDist_Tag] -> run_SWC_FDC_RxTx_5ms_sys/59(IRV_u8Array8_PasInDist_read)
  run_SWC_FDC_Tx_10ms_sys/15(IRV_u8Array8_ApsInLevel_write) -> [IRV_u8Array8_ApsInLevel_Tag]  "IRV_u8Array8_ApsInLevel"
  [IRV_u8Array8_ApsInLevel_Tag] -> run_SWC_FDC_RxTx_5ms_sys/58(IRV_u8Array8_ApsInLevel_read)
  run_SWC_FDC_Tx_10ms_sys/14(IRV_u8Array12_ApsInUssSta_write) -> [IRV_u8Array12_ApsInUssSta_Tag]  "IRV_u8Array12_ApsInUssSta"
  [IRV_u8Array12_ApsInUssSta_Tag] -> run_SWC_FDC_RxTx_5ms_sys/56(IRV_u8Array12_ApsInUssSta_read)
  run_SWC_FDC_Tx_10ms_sys/13(IRV_u16Array4_ApsInDist_write) -> [IRV_u16Array4_ApsInDist_Tag]  "IRV_u16Array4_ApsInDist"
  [IRV_u16Array4_ApsInDist_Tag] -> run_SWC_FDC_RxTx_5ms_sys/55(IRV_u16Array4_ApsInDist_read)
  run_SWC_FDC_PAS_1ms/1 -> run_SWC_FDC_PAS_1ms_sys/Trigger
  run_SWC_FDC_UDS_10ms/1 -> run_SWC_FDC_UDS_10ms_sys/Trigger
  run_SWC_FDC_CDD_10ms/1 -> run_SWC_FDC_CDD_10ms_sys/Trigger
  run_SWC_FDC_RxTx_5ms/1 -> run_SWC_FDC_RxTx_5ms_sys/Trigger
  run_SWC_FDC_Tx_10ms/1 -> run_SWC_FDC_Tx_10ms_sys/Trigger
  run_SWC_FDC_Tx_5000ms/1 -> run_SWC_FDC_Tx_5000ms_sys/Trigger
  run_SWC_FDC_Tx_500ms/1 -> run_SWC_FDC_Tx_500ms_sys/Trigger
  run_SWC_FDC_Tx_20ms/1 -> run_SWC_FDC_Tx_20ms_sys/Trigger
  run_SWC_FDC_Tx_1000ms/1 -> run_SWC_FDC_Tx_1000ms_sys/Trigger
  run_SWC_FDC_Tx_100ms/1 -> run_SWC_FDC_Tx_100ms_sys/Trigger
  R_CAN4_zGW_LINDr2_CAN4_SG_zGW_LINDr2/1 -> run_SWC_FDC_RxTx_5ms_sys/77(R_CAN4_zGW_LINDr2_CAN4_SG_zGW_LINDr2_read)
  R_CAN4_zGW_LINFr2_CAN4_SG_zGW_LINFr2/1 -> run_SWC_FDC_RxTx_5ms_sys/78(R_CAN4_zGW_LINFr2_CAN4_SG_zGW_LINFr2_read)
  R_CAN6_FCM2_CAN6_SG_FCM2/1 -> run_SWC_FDC_RxTx_5ms_sys/79(R_CAN6_FCM2_CAN6_SG_FCM2_read)
  R_CAN4_BodyZone_DR2_CAN4_SG_BodyZone_DR2/1 -> run_SWC_FDC_RxTx_5ms_sys/80(R_CAN4_BodyZone_DR2_CAN4_SG_BodyZone_DR2_read)

== system SWC_FDC_type/P_WDGCDD ==
  run_SWC_FDC_AppCallWDG_End_sys : Subsystem
  run_SWC_FDC_AppCallWDG_StartUp_sys : Subsystem
  run_SWC_FDC_AppCallWDG_sys : Subsystem

== system SWC_FDC_type/SWC_FDC_type_Init ==
  Event Listener : EventListener  EventName=reset

== system SWC_FDC_type/run_SWC_FDC_AppCallSleep_sys ==
  function : TriggerPort  TriggerType=function-call  IsSimulinkFunction=on  FunctionName=run_SWC_FDC_AppCallSleep  VariantControl=(inherit)
  Constant : Constant  Value=TRUE
  Data Type Conversion : DataTypeConversion  OutDataTypeStr=Enum: AppModeRequestType
  Data Type Conversion1 : DataTypeConversion  OutDataTypeStr=uint8
  P_AppModeReq_requestedMode_write : Outport
  wires:
  Data Type Conversion/1 -> P_AppModeReq_requestedMode_write/1
  Data Type Conversion1/1 -> Data Type Conversion/1
  Constant/1 -> Data Type Conversion1/1

== system SWC_FDC_type/run_SWC_FDC_CDD_10ms_sys ==
  function : TriggerPort  TriggerType=function-call  VariantControl=(inherit)  SampleTimeType=periodic  SampleTime=-1
  R_HALINCDD_CSOP_HALINCDD_IOEXPANDER : FunctionCaller  FunctionPrototype=[u8_HoodSW,u8_TailgateSW,u8_DrDoorSW,u8_PsDoorSW,u8_RRDoorSW,u8_RLDoorSW,u8_CTDSW,u8_HazardSW,u8_TrunkHanSW,u8_SeatSW,u8_CrashSignal] = R_HALINCDD_CSOP_HALINCDD_IOEXPANDER()  OutputArgumentSpecifications=uint8(1), uint8(1), uint8(1), uint8(1), uint8(1), uint8(1), uint8(1), uint8(1), uint8(1), uint8(1), uint8(1)
  IRV_u8_CTDSW_write : Outport  OutDataTypeStr=uint8  PortDimensions=1
  IRV_u8_CrashSignal_write : Outport  Port=2  OutDataTypeStr=uint8  PortDimensions=1
  IRV_u8_DrDoorSW_write : Outport  Port=3  OutDataTypeStr=uint8  PortDimensions=1
  IRV_u8_HazardSW_write : Outport  Port=4  OutDataTypeStr=uint8  PortDimensions=1
  IRV_u8_HoodSW_write : Outport  Port=5  OutDataTypeStr=uint8  PortDimensions=1
  IRV_u8_PsDoorSW_write : Outport  Port=6  OutDataTypeStr=uint8  PortDimensions=1
  IRV_u8_RLDoorSW_write : Outport  Port=7  OutDataTypeStr=uint8  PortDimensions=1
  IRV_u8_RRDoorSW_write : Outport  Port=8  OutDataTypeStr=uint8  PortDimensions=1
  IRV_u8_SeatSW_write : Outport  Port=9  OutDataTypeStr=uint8  PortDimensions=1
  IRV_u8_TailgateSW_write : Outport  Port=10  OutDataTypeStr=uint8  PortDimensions=1
  IRV_u8_TrunkHanSW_write : Outport  Port=11  OutDataTypeStr=uint8  PortDimensions=1
  wires:
  R_HALINCDD_CSOP_HALINCDD_IOEXPANDER/1 -> IRV_u8_HoodSW_write/1
  R_HALINCDD_CSOP_HALINCDD_IOEXPANDER/2 -> IRV_u8_TailgateSW_write/1
  R_HALINCDD_CSOP_HALINCDD_IOEXPANDER/3 -> IRV_u8_DrDoorSW_write/1
  R_HALINCDD_CSOP_HALINCDD_IOEXPANDER/4 -> IRV_u8_PsDoorSW_write/1
  R_HALINCDD_CSOP_HALINCDD_IOEXPANDER/5 -> IRV_u8_RRDoorSW_write/1
  R_HALINCDD_CSOP_HALINCDD_IOEXPANDER/6 -> IRV_u8_RLDoorSW_write/1
  R_HALINCDD_CSOP_HALINCDD_IOEXPANDER/7 -> IRV_u8_CTDSW_write/1
  R_HALINCDD_CSOP_HALINCDD_IOEXPANDER/8 -> IRV_u8_HazardSW_write/1
  R_HALINCDD_CSOP_HALINCDD_IOEXPANDER/9 -> IRV_u8_TrunkHanSW_write/1
  R_HALINCDD_CSOP_HALINCDD_IOEXPANDER/10 -> IRV_u8_SeatSW_write/1
  R_HALINCDD_CSOP_HALINCDD_IOEXPANDER/11 -> IRV_u8_CrashSignal_write/1

== system SWC_FDC_type/run_SWC_FDC_E2E_Write_CAN3VCU1_sys ==
  IRV_E2E_CAN3_SG_FD3_VCU1_read : Inport
  function : TriggerPort  TriggerType=function-call  IsSimulinkFunction=on  FunctionName=run_SWC_FDC_E2E_Write_CAN3VCU1  VariantControl=(inherit)
  P_CAN3_FD3_VCU1_CAN3_SG_FD3_VCU1_write : Outport
  wires:
  IRV_E2E_CAN3_SG_FD3_VCU1_read/1 -> P_CAN3_FD3_VCU1_CAN3_SG_FD3_VCU1_write/1

== system SWC_FDC_type/run_SWC_FDC_E2E_Write_CAN3VCU1_toNIDEC_sys ==
  IRV_E2E_CAN3_SG_FD3_VCU1_toNIDEC_read : Inport
  function : TriggerPort  TriggerType=function-call  IsSimulinkFunction=on  FunctionName=run_SWC_FDC_E2E_Write_CAN3VCU1_toNIDEC  VariantControl=(inherit)
  P_CAN3_FD3_VCU1_toNIDEC_CAN3_SG_FD3_VCU1_toNIDEC_write : Outport
  wires:
  IRV_E2E_CAN3_SG_FD3_VCU1_toNIDEC_read/1 -> P_CAN3_FD3_VCU1_toNIDEC_CAN3_SG_FD3_VCU1_toNIDEC_write/1

== system SWC_FDC_type/run_SWC_FDC_E2E_Write_CAN4VCU1_sys ==
  IRV_E2E_CAN4_SG_FD4_CE100_0_read : Inport
  function : TriggerPort  TriggerType=function-call  IsSimulinkFunction=on  FunctionName=run_SWC_FDC_E2E_Write_CAN4VCU1  VariantControl=(inherit)
  P_CAN4_FD4_CE100_0_CAN4_SG_FD4_CE100_0_write : Outport
  wires:
  IRV_E2E_CAN4_SG_FD4_CE100_0_read/1 -> P_CAN4_FD4_CE100_0_CAN4_SG_FD4_CE100_0_write/1

== system SWC_FDC_type/run_SWC_FDC_NvmRead_sys ==
  R_NVMRead_NV_FVTDataArray_read : Inport
  function : TriggerPort  TriggerType=function-call  IsSimulinkFunction=on  FunctionName=run_SWC_FDC_NvmRead  VariantControl=(inherit)
  IRV_u8Array256_NvmReadArray_write : Outport  OutDataTypeStr=uint8  PortDimensions=256
  wires:
  R_NVMRead_NV_FVTDataArray_read/1 -> IRV_u8Array256_NvmReadArray_write/1

== system SWC_FDC_type/run_SWC_FDC_NvmWrite_sys ==
  IRV_u8Array256_NvmWriteArray_read : Inport
  function : TriggerPort  TriggerType=function-call  IsSimulinkFunction=on  FunctionName=run_SWC_FDC_NvmWrite  VariantControl=(inherit)
  P_NVMWrite_NV_FVTDataArray_write : Outport
  wires:
  IRV_u8Array256_NvmWriteArray_read/1 -> P_NVMWrite_NV_FVTDataArray_write/1

== system SWC_FDC_type/run_SWC_FDC_PAS_1ms_sys ==
  function : TriggerPort  TriggerType=function-call  VariantControl=(inherit)  SampleTimeType=periodic  SampleTime=-1
  R_HALINCDD_CSOP_PAS_Handler : FunctionCaller  FunctionPrototype=R_HALINCDD_CSOP_PAS_Handler()
